simulink model "TestCommandGenerator"  (R2021b)
settings: Solver=VariableStepAuto  StartTime=0.0  StopTime=20  RelTol=1e-3
values from neighbouring files (symbols this model uses):
  A = [(q1^2 - q2^2 - q3^2 + q4^2), 2*(q1*q2 + q3*q4), 2*(q1*q3 - q2*q4);            2*(q1*q2 - q3*q4), (-q1^2 + q2^2 - q3^2 + q4^2), 2*(q2*q3 + q1*q4);            2*(q1*q3 + q2*q4), 2*(q2*q3 - q1*q4), (-q1^2 - q2^2 + q3^2 + q4^2)]    [RunCommandGenerator.m]
  C = 1/cos(theta)*[0 sin(phi) cos(phi); 0 cos(phi)*cos(theta) -sin(phi)*cos(theta); cos(theta) sin(phi)*sin(theta) cos(phi)*sin(theta)]    [InverseKinematics.m]
  phi = zeros(length(q),1)    [RunCommandGenerator.m]
  psi = phi    [RunCommandGenerator.m]
  theta = phi    [RunCommandGenerator.m]
undefined symbols (not defined in the file or in its folder): B, D
settings Model: Creator=17165  LastModifiedBy=17165

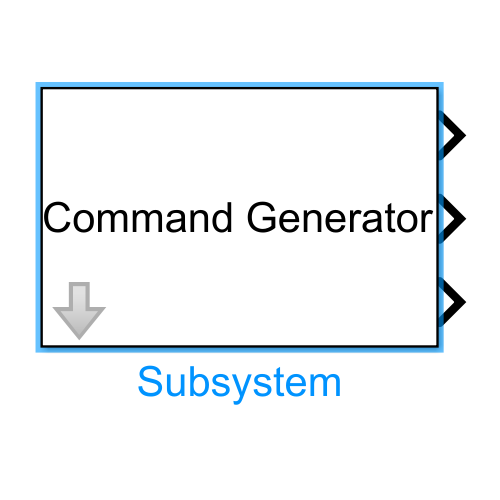
[thumbnail: Simulink's stored preview of the top-level diagram]
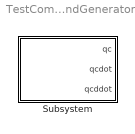
== system TestCommandGenerator ==
  Subsystem : Subsystem  mask{A=A, B=B, C=C, D=D, phic=phi, thetac=theta, psic=psi}
      mask prompts: A "Filter A"; B "FIlter B"; C "FIlter C"; D "Filter C"; phic "Roll command"; thetac "Pitch command"; psic "Roll command"
      mask Display: disp('Command Generator')

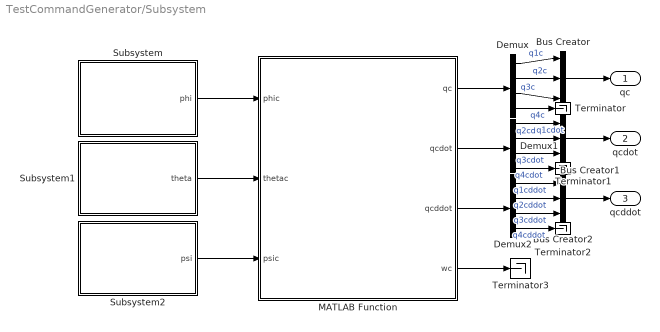
== system TestCommandGenerator/Subsystem ==
  Bus Creator : BusCreator  Inputs=3
  Bus Creator1 : BusCreator  Inputs=3
  Bus Creator2 : BusCreator  Inputs=3
  Demux : Demux
  Demux1 : Demux
  Demux2 : Demux
  MATLAB Function : MATLAB Function  TreatAsAtomicUnit=on
  Subsystem : Subsystem  mask{A=A, B=B, C=C, D=D, amp=phic}
      mask prompts: A "FIlter A Matrix"; B "Filter B Matrix"; C "Filter C Matrix"; D "Filter D Matrix"; amp "Quaternion Command"
      mask Display: disp('Filtered Command')
  Subsystem1 : Subsystem  mask{A=A, B=B, C=C, D=D, amp=thetac}
      mask prompts: A "FIlter A Matrix"; B "Filter B Matrix"; C "Filter C Matrix"; D "Filter D Matrix"; amp "Quaternion Command"
      mask Display: disp('Filtered Command')
  Subsystem2 : Subsystem  mask{A=A, B=B, C=C, D=D, amp=psic}
      mask prompts: A "FIlter A Matrix"; B "Filter B Matrix"; C "Filter C Matrix"; D "Filter D Matrix"; amp "Quaternion Command"
      mask Display: disp('Filtered Command')
  Terminator{,1..3} (4 alike) : Terminator
  qc : Outport
  qcdot : Outport  Port=2
  qcddot : Outport  Port=3
  wires:
  Subsystem/1(phi) -> MATLAB Function/1(phic)
  Subsystem1/1(theta) -> MATLAB Function/2(thetac)
  Subsystem2/1(psi) -> MATLAB Function/3(psic)
  MATLAB Function/2(qcdot) -> Demux1/1
  MATLAB Function/1(qc) -> Demux/1
  MATLAB Function/4(wc) -> Terminator3/1
  Demux/1 -> Bus Creator/1  "q1c"
  Demux/2 -> Bus Creator/2  "q2c"
  Demux/3 -> Bus Creator/3  "q3c"
  Demux/4 -> Terminator/1  "q4c"
  Bus Creator/1 -> qc/1
  Demux1/2 -> Bus Creator1/2  "q2cdot"
  Bus Creator1/1 -> qcdot/1
  Demux1/1 -> Bus Creator1/1  "q1cdot"
  Demux1/3 -> Bus Creator1/3  "q3cdot"
  Demux1/4 -> Terminator1/1  "q4cdot"
  Bus Creator2/1 -> qcddot/1
  MATLAB Function/3(qcddot) -> Demux2/1
  Demux2/1 -> Bus Creator2/1  "q1cddot"
  Demux2/2 -> Bus Creator2/2  "q2cddot"
  Demux2/3 -> Bus Creator2/3  "q3cddot"
  Demux2/4 -> Terminator2/1  "q4cddot"

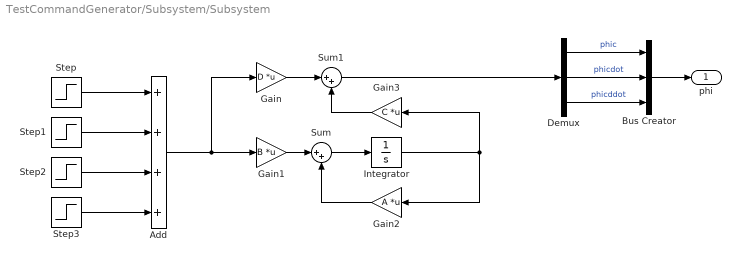
== system TestCommandGenerator/Subsystem/Subsystem ==
  Add : Sum  Inputs=++++
  Bus Creator : BusCreator  Inputs=3
  Demux : Demux  Outputs=3
  Gain : Gain  Gain=D  Multiplication=Matrix(K*u)
  Gain1 : Gain  Gain=B  Multiplication=Matrix(K*u)
  Gain2 : Gain  Gain=A  Multiplication=Matrix(K*u)
  Gain3 : Gain  Gain=C  Multiplication=Matrix(K*u)
  Integrator : Integrator
  Step : Step  After=amp  SampleTime=0
  Step1 : Step  Time=6  After=-amp  SampleTime=0
  Step2 : Step  Time=6  After=-amp  SampleTime=0
  Step3 : Step  Time=11  After=amp  SampleTime=0
  Sum : Sum  Inputs=|++
  Sum1 : Sum  Inputs=|++
  phi : Outport
  wires:
  Gain/1 -> Sum1/1
  Sum1/1 -> Demux/1
  Add/1 -> Gain/1, Gain1/1
  Step2/1 -> Add/3
  Gain1/1 -> Sum/1
  Integrator/1 -> Gain2/1, Gain3/1
  Step1/1 -> Add/2
  Step/1 -> Add/1
  Gain3/1 -> Sum1/2
  Step3/1 -> Add/4
  Gain2/1 -> Sum/2
  Sum/1 -> Integrator/1
  Bus Creator/1 -> phi/1
  Demux/1 -> Bus Creator/1  "phic"
  Demux/2 -> Bus Creator/2  "phicdot"
  Demux/3 -> Bus Creator/3  "phicddot"

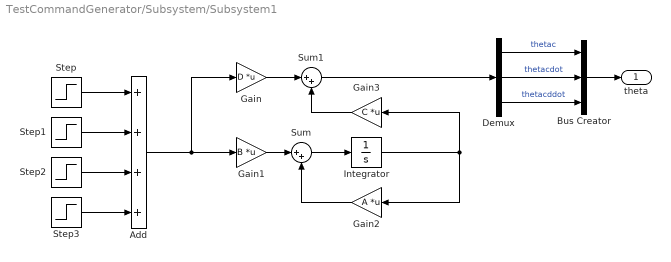
== system TestCommandGenerator/Subsystem/Subsystem1 ==
  Add : Sum  Inputs=++++
  Bus Creator : BusCreator  Inputs=3
  Demux : Demux  Outputs=3
  Gain : Gain  Gain=D  Multiplication=Matrix(K*u)
  Gain1 : Gain  Gain=B  Multiplication=Matrix(K*u)
  Gain2 : Gain  Gain=A  Multiplication=Matrix(K*u)
  Gain3 : Gain  Gain=C  Multiplication=Matrix(K*u)
  Integrator : Integrator
  Step : Step  After=amp  SampleTime=0
  Step1 : Step  Time=6  After=-amp  SampleTime=0
  Step2 : Step  Time=6  After=-amp  SampleTime=0
  Step3 : Step  Time=11  After=amp  SampleTime=0
  Sum : Sum  Inputs=|++
  Sum1 : Sum  Inputs=|++
  theta : Outport
  wires:
  Gain/1 -> Sum1/1
  Add/1 -> Gain/1, Gain1/1
  Step2/1 -> Add/3
  Gain1/1 -> Sum/1
  Integrator/1 -> Gain2/1, Gain3/1
  Step1/1 -> Add/2
  Step/1 -> Add/1
  Gain3/1 -> Sum1/2
  Step3/1 -> Add/4
  Gain2/1 -> Sum/2
  Sum/1 -> Integrator/1
  Demux/3 -> Bus Creator/3  "thetacddot"
  Demux/1 -> Bus Creator/1  "thetac"
  Sum1/1 -> Demux/1
  Bus Creator/1 -> theta/1
  Demux/2 -> Bus Creator/2  "thetacdot"

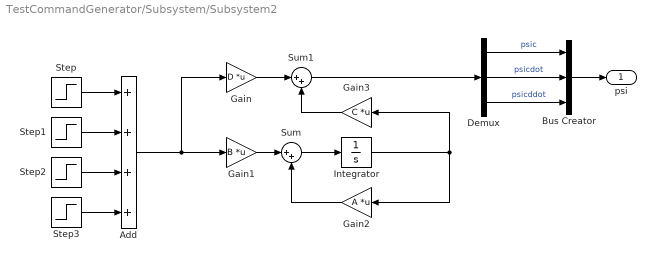
== system TestCommandGenerator/Subsystem/Subsystem2 ==
  Add : Sum  Inputs=++++
  Bus Creator : BusCreator  Inputs=3
  Demux : Demux  Outputs=3
  Gain : Gain  Gain=D  Multiplication=Matrix(K*u)
  Gain1 : Gain  Gain=B  Multiplication=Matrix(K*u)
  Gain2 : Gain  Gain=A  Multiplication=Matrix(K*u)
  Gain3 : Gain  Gain=C  Multiplication=Matrix(K*u)
  Integrator : Integrator
  Step : Step  After=amp  SampleTime=0
  Step1 : Step  Time=6  After=-amp  SampleTime=0
  Step2 : Step  Time=6  After=-amp  SampleTime=0
  Step3 : Step  Time=11  After=amp  SampleTime=0
  Sum : Sum  Inputs=|++
  Sum1 : Sum  Inputs=|++
  psi : Outport
  wires:
  Gain/1 -> Sum1/1
  Add/1 -> Gain/1, Gain1/1
  Step2/1 -> Add/3
  Gain1/1 -> Sum/1
  Integrator/1 -> Gain2/1, Gain3/1
  Step1/1 -> Add/2
  Step/1 -> Add/1
  Gain3/1 -> Sum1/2
  Step3/1 -> Add/4
  Gain2/1 -> Sum/2
  Sum/1 -> Integrator/1
  Demux/3 -> Bus Creator/3  "psicddot"
  Demux/1 -> Bus Creator/1  "psic"
  Sum1/1 -> Demux/1
  Bus Creator/1 -> psi/1
  Demux/2 -> Bus Creator/2  "psicdot"

== matlab function TestCommandGenerator/Subsystem/MATLAB Function ==
  data: phic input; thetac input; psic input; qc output; qcdot output; qcddot output; wc output
function [qc,qcdot, qcddot, wc] = QuaternionCommandGenerator(phic,thetac,psic)
qc      = zeros(4,1);
qcdot   = zeros(4,1);
qcddot  = zeros(4,1);
[qc,qcdot, qcddot, wc] = QuaternionCommand(phic,thetac,psic);


end
